simulink model "DiscreteTesting"  (R2018b)
settings: Solver=VariableStepAuto  StartTime=0.0  StopTime=200  RelTol=1e-3
libraries: fuzblock x1
settings Model: Creator=soren  LastModifiedBy=soren

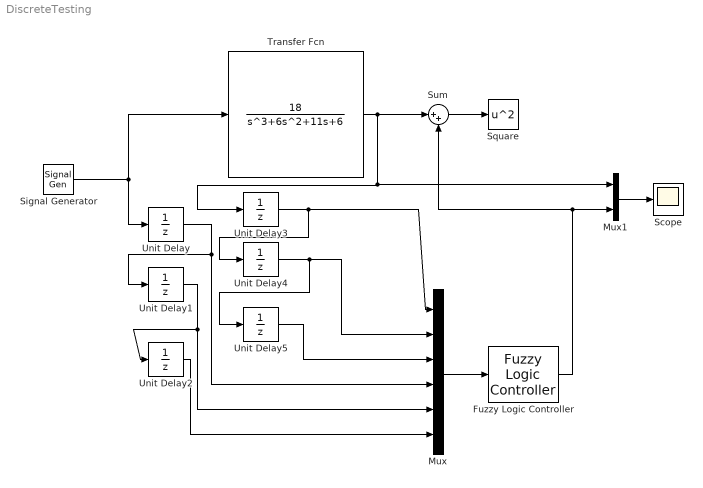
== system DiscreteTesting ==
  Fuzzy Logic Controller : fuzblock/Fuzzy Logic  Controller  FIS=fis4  OutputSampleNumber=101  DataType=double  FuzzifiedInputs=off  RuleFiringStrengths=off  RuleOutputs=off  AggregatedOutputs=off  SimulateUsing=Interpreted execution  OutOfRangeInputValueMessage=warning  NoRuleFiredMessage=warning  EmptyOutputFuzzySetMessage=warning
  Mux : Mux  Inputs=6
  Mux1 : Mux  Inputs=2
  Scope : Scope
  Signal Generator : SignalGenerator  Frequency=0.1  Units=rad/sec
  Square : Math  Operator=square  RndMeth=Zero  SaturateOnIntegerOverflow=on
  Sum : Sum  Inputs=|++
  Transfer Fcn : TransferFcn  Numerator=[18]  Denominator=[1 6 11 6]
  Unit Delay{,1..5} (6 alike) : UnitDelay  SampleTime=0.03
  wires:
  Signal Generator/1 -> Unit Delay/1, Transfer Fcn/1
  Unit Delay/1 -> Mux/4, Unit Delay1/1
  Unit Delay1/1 -> Mux/5, Unit Delay2/1
  Unit Delay4/1 -> Mux/2, Unit Delay5/1
  Unit Delay3/1 -> Unit Delay4/1, Mux/1
  Transfer Fcn/1 -> Sum/1, Unit Delay3/1, Mux1/1
  Mux/1 -> Fuzzy Logic Controller/1
  Unit Delay5/1 -> Mux/3
  Unit Delay2/1 -> Mux/6
  Mux1/1 -> Scope/1
  Fuzzy Logic Controller/1 -> Sum/2, Mux1/2
  Sum/1 -> Square/1
